simulink model "RO_Plantsimscape"  (R2020a)
settings: Solver=VariableStepAuto  StartTime=0.0  StopTime=100  RelTol=1e-3
libraries: sh_lib x108, fl_lib x76, nesl_utility x73, simulink x13
(part 4 of 4)

== system RO_Plantsimscape/PSOC8 ==
  E : Inport
  Hydraulic Flow Rate Sensor : fl_lib/Hydraulic/Hydraulic Sensors/Hydraulic Flow Rate Sensor
  PS-Simulink Converter2 : nesl_utility/PS-Simulink Converter  PhysicalDomain=network_engine_domain  SubClassName=ps_output  LeftPortType=input  RightPortType=output  PseudoPeriodic=off  Frequencies=[]  Unit=1  AffineConversion=off
  Pipe P : sh_lib/Low-Pressure Blocks/Resistive Pipe LP  cs_type=1  d_in=112.1660 mm  area=1e-04 m^2  D_h=0.0112 m  s_factor=64  length=8.1 m  length_ad=1 m  roughness=0.005 mm  Re_lam=2e+03  Re_turb=4e+03  elevation_A=45 m  elevation_B=45 m  g=9.80665 m/s^2  pressure_drop_specify=off  pressure_drop_priority=None  pressure_drop=0 Pa  pressure_drop_nominal_specify=off  pressure_drop_nominal_unit=Pa  pressure_drop_nominal_value=1  flow_rate_specify=off  flow_rate_priority=None  flow_rate=0 m^3/s  flow_rate_nominal_specify=off  flow_rate_nominal_unit=m^3/s  flow_rate_nominal_value=1
      settings: SourceProductBaseCode=SH  InternalSimscapePortConfiguration="{\"Bottom\":[],\"Left\":[{\"id\":\"A\",\"label\":\"A\",\"type\":\"foundation.hydraulic.hydraulic\"}],\"Right\":[{\"id\":\"B\",\"label\":\"B\",\"type\":\"foundation.hydraulic.hydraulic\"}],\"Top\":[]}"
  "Pneumatic Pump, Drive and Amplifier" : TransferFcn  Denominator=[0.1 1]
  Poppet Valve : sh_lib/Valves/Flow Control Valves/Poppet Valve  d_stem=0.01 m  cone_angle=120 deg  x_0=0 m  C_d=0.65  A_leak=1e-12 m^2  lam_spec=1  B_lam=0.999  Re_cr=10
      settings: SourceProductBaseCode=SH  InternalSimscapePortConfiguration="{\"Bottom\":[],\"Left\":[{\"id\":\"S\",\"label\":\"S\",\"type\":\"input\"},{\"id\":\"A\",\"label\":\"A\",\"type\":\"foundation.hydraulic.hydraulic\"}],\"Right\":[{\"id\":\"B\",\"label\":\"B\",\"type\":\"foundation.hydraulic.hydraulic\"}],\"Top\":[]}"
  Saturation : Saturate  UpperLimit=100  LowerLimit=0
  Scope : Scope
  Scope1 : Scope
  Simulink-PS Converter1 : nesl_utility/Simulink-PS Converter  PhysicalDomain=network_engine_domain  SubClassName=ps_input  LeftPortType=input  RightPortType=output  PseudoPeriodic=off  Frequencies=[]  NoiseDistribution=none  NoiseParameters=[]  Unit=1  AffineConversion=on  FilteringAndDerivatives=zero  SimscapeFilterOrder=1  InputFilterTimeConstant=.001  UdotUserProvided=0
  Valve Stiction : TransportDelay  DelayTime=0.5
  Out : PMIOPort  Side=Right
  In : PMIOPort  Port=2  Side=Left
  wires:
  E/1 -> "Pneumatic Pump, Drive and Amplifier"/1
  "Pneumatic Pump, Drive and Amplifier"/1 -> Valve Stiction/1
  PS-Simulink Converter2/1 -> Scope1/1
  Valve Stiction/1 -> Saturation/1
  Saturation/1 -> Scope/1, Simulink-PS Converter1/1
  connections:
  Simulink-PS Converter1/RConn1 -- Poppet Valve/LConn1
  In/RConn1 -- Poppet Valve/LConn2
  Hydraulic Flow Rate Sensor/RConn2 -- Out/RConn1
  Hydraulic Flow Rate Sensor/RConn1 -- PS-Simulink Converter2/LConn1
  Poppet Valve/RConn1 -- Pipe P/LConn1
  Hydraulic Flow Rate Sensor/LConn1 -- Pipe P/RConn1

== system RO_Plantsimscape/PSOC9 ==
  E : Inport
  Hydraulic Flow Rate Sensor : fl_lib/Hydraulic/Hydraulic Sensors/Hydraulic Flow Rate Sensor
  PS-Simulink Converter2 : nesl_utility/PS-Simulink Converter  PhysicalDomain=network_engine_domain  SubClassName=ps_output  LeftPortType=input  RightPortType=output  PseudoPeriodic=off  Frequencies=[]  Unit=1  AffineConversion=off
  Pipe P : sh_lib/Low-Pressure Blocks/Resistive Pipe LP  cs_type=1  d_in=112.1660 mm  area=1e-04 m^2  D_h=0.0112 m  s_factor=64  length=8.1 m  length_ad=1 m  roughness=0.005 mm  Re_lam=2e+03  Re_turb=4e+03  elevation_A=45 m  elevation_B=45 m  g=9.80665 m/s^2  pressure_drop_specify=off  pressure_drop_priority=None  pressure_drop=0 Pa  pressure_drop_nominal_specify=off  pressure_drop_nominal_unit=Pa  pressure_drop_nominal_value=1  flow_rate_specify=off  flow_rate_priority=None  flow_rate=0 m^3/s  flow_rate_nominal_specify=off  flow_rate_nominal_unit=m^3/s  flow_rate_nominal_value=1
      settings: SourceProductBaseCode=SH  InternalSimscapePortConfiguration="{\"Bottom\":[],\"Left\":[{\"id\":\"A\",\"label\":\"A\",\"type\":\"foundation.hydraulic.hydraulic\"}],\"Right\":[{\"id\":\"B\",\"label\":\"B\",\"type\":\"foundation.hydraulic.hydraulic\"}],\"Top\":[]}"
  "Pneumatic Pump, Drive and Amplifier" : TransferFcn  Denominator=[0.1 1]
  Poppet Valve : sh_lib/Valves/Flow Control Valves/Poppet Valve  d_stem=0.01 m  cone_angle=120 deg  x_0=0 m  C_d=0.65  A_leak=1e-12 m^2  lam_spec=1  B_lam=0.999  Re_cr=10
      settings: SourceProductBaseCode=SH  InternalSimscapePortConfiguration="{\"Bottom\":[],\"Left\":[{\"id\":\"S\",\"label\":\"S\",\"type\":\"input\"},{\"id\":\"A\",\"label\":\"A\",\"type\":\"foundation.hydraulic.hydraulic\"}],\"Right\":[{\"id\":\"B\",\"label\":\"B\",\"type\":\"foundation.hydraulic.hydraulic\"}],\"Top\":[]}"
  Saturation : Saturate  UpperLimit=100  LowerLimit=0
  Scope : Scope
  Scope1 : Scope
  Simulink-PS Converter1 : nesl_utility/Simulink-PS Converter  PhysicalDomain=network_engine_domain  SubClassName=ps_input  LeftPortType=input  RightPortType=output  PseudoPeriodic=off  Frequencies=[]  NoiseDistribution=none  NoiseParameters=[]  Unit=1  AffineConversion=on  FilteringAndDerivatives=zero  SimscapeFilterOrder=1  InputFilterTimeConstant=.001  UdotUserProvided=0
  Valve Stiction : TransportDelay  DelayTime=0.5
  Out : PMIOPort  Side=Right
  In : PMIOPort  Port=2  Side=Left
  wires:
  E/1 -> "Pneumatic Pump, Drive and Amplifier"/1
  "Pneumatic Pump, Drive and Amplifier"/1 -> Valve Stiction/1
  PS-Simulink Converter2/1 -> Scope1/1
  Valve Stiction/1 -> Saturation/1
  Saturation/1 -> Scope/1, Simulink-PS Converter1/1
  connections:
  Simulink-PS Converter1/RConn1 -- Poppet Valve/LConn1
  In/RConn1 -- Poppet Valve/LConn2
  Hydraulic Flow Rate Sensor/RConn2 -- Out/RConn1
  Hydraulic Flow Rate Sensor/RConn1 -- PS-Simulink Converter2/LConn1
  Poppet Valve/RConn1 -- Pipe P/LConn1
  Hydraulic Flow Rate Sensor/LConn1 -- Pipe P/RConn1

== system RO_Plantsimscape/Rain ==
  Centrifugal Pump : Subsystem
      mask Display: image('$imagefile'); % Use "Edit Image" on toolstrip to change.
  Constant4 : Constant  Value=3000
  Poppet Valve : sh_lib/Valves/Flow Control Valves/Poppet Valve  d_stem=1 m  cone_angle=120 deg  x_0=0 m  C_d=1  A_leak=1e-12 m^2  lam_spec=2  B_lam=0.999  Re_cr=2300
      settings: SourceProductBaseCode=SH  InternalSimscapePortConfiguration="{\"Bottom\":[],\"Left\":[{\"id\":\"S\",\"label\":\"S\",\"type\":\"input\"},{\"id\":\"A\",\"label\":\"A\",\"type\":\"foundation.hydraulic.hydraulic\"}],\"Right\":[{\"id\":\"B\",\"label\":\"B\",\"type\":\"foundation.hydraulic.hydraulic\"}],\"Top\":[]}"
  Rain : sh_lib/Low-Pressure Blocks/Constant Head Tank  press=1 Pa  fluid_level=10000 m  pipe_diam=0.02 m  loss_coeff=1.2  g=9.80665 m/s^2  volume_specify=on  volume_priority=High  volume=1000 m^3  volume_nominal_specify=off  volume_nominal_unit=m^3  volume_nominal_value=1
      settings: SourceProductBaseCode=SH  InternalSimscapePortConfiguration="{\"Bottom\":[],\"Left\":[],\"Right\":[{\"id\":\"V\",\"label\":\"V\",\"type\":\"output\"},{\"id\":\"T\",\"label\":\"T\",\"type\":\"foundation.hydraulic.hydraulic\"}],\"Top\":[]}"
  Simulink-PS Converter1 : nesl_utility/Simulink-PS Converter  PhysicalDomain=network_engine_domain  SubClassName=ps_input  LeftPortType=input  RightPortType=output  PseudoPeriodic=off  Frequencies=[]  NoiseDistribution=none  NoiseParameters=[]  Unit=1  AffineConversion=on  FilteringAndDerivatives=zero  SimscapeFilterOrder=1  InputFilterTimeConstant=.001  UdotUserProvided=0
  Sine Wave : Sin  Amplitude=10  Frequency=0.5  SampleTime=0
  Rain_ : PMIOPort  Side=Right
  wires:
  Sine Wave/1 -> Simulink-PS Converter1/1
  Constant4/1 -> Centrifugal Pump/1(f)
  connections:
  Poppet Valve/LConn1 -- Simulink-PS Converter1/RConn1
  Rain_/RConn1 -- Poppet Valve/RConn1
  Centrifugal Pump/LConn1 -- Rain/RConn2
  Centrifugal Pump/RConn1 -- Poppet Valve/LConn2

== system RO_Plantsimscape/Centrifugal Pump1/induction machine ==
  note: Voltage/Hz control
  note: TODO: Set the number of poles,
      | the induction machine's time constant and
      | the maximum rotor speed in rad/s
  f : Inport
  Induction Machine : TransferFcn  Denominator=[1 1]
  Induction speed : MATLAB Function  TreatAsAtomicUnit=on
  max/min speeds : Saturate  UpperLimit=100  LowerLimit=0
  w : Outport
  wires:
  f/1 -> Induction speed/1(f)
  Induction speed/1(w) -> Induction Machine/1
  max/min speeds/1 -> w/1
  Induction Machine/1 -> max/min speeds/1

== system RO_Plantsimscape/Centrifugal Pump2/induction machine ==
  note: Voltage/Hz control
  note: TODO: Set the number of poles,
      | the induction machine's time constant and
      | the maximum rotor speed in rad/s
  f : Inport
  Induction Machine : TransferFcn  Denominator=[1 1]
  Induction speed : MATLAB Function  TreatAsAtomicUnit=on
  max/min speeds : Saturate  UpperLimit=10000  LowerLimit=0
  w : Outport
  wires:
  f/1 -> Induction speed/1(f)
  Induction speed/1(w) -> Induction Machine/1
  max/min speeds/1 -> w/1
  Induction Machine/1 -> max/min speeds/1

== system RO_Plantsimscape/Centrifugal Pump3/induction machine ==
  note: Voltage/Hz control
  note: TODO: Set the number of poles,
      | the induction machine's time constant and
      | the maximum rotor speed in rad/s
  f : Inport
  Induction Machine : TransferFcn  Denominator=[1 1]
  Induction speed : MATLAB Function  TreatAsAtomicUnit=on
  max/min speeds : Saturate  UpperLimit=10000  LowerLimit=0
  w : Outport
  wires:
  f/1 -> Induction speed/1(f)
  Induction speed/1(w) -> Induction Machine/1
  max/min speeds/1 -> w/1
  Induction Machine/1 -> max/min speeds/1

== system RO_Plantsimscape/Centrifugal Pump4/induction machine ==
  note: Voltage/Hz control
  note: TODO: Set the number of poles,
      | the induction machine's time constant and
      | the maximum rotor speed in rad/s
  f : Inport
  Induction Machine : TransferFcn  Denominator=[1 1]
  Induction speed : MATLAB Function  TreatAsAtomicUnit=on
  max/min speeds : Saturate  UpperLimit=10000  LowerLimit=0
  w : Outport
  wires:
  f/1 -> Induction speed/1(f)
  Induction speed/1(w) -> Induction Machine/1
  max/min speeds/1 -> w/1
  Induction Machine/1 -> max/min speeds/1

== system RO_Plantsimscape/Centrifugal Pump5/induction machine ==
  note: Voltage/Hz control
  note: TODO: Set the number of poles,
      | the induction machine's time constant and
      | the maximum rotor speed in rad/s
  f : Inport
  Induction Machine : TransferFcn  Denominator=[1 1]
  Induction speed : MATLAB Function  TreatAsAtomicUnit=on
  max/min speeds : Saturate  UpperLimit=100  LowerLimit=0
  w : Outport
  wires:
  f/1 -> Induction speed/1(f)
  Induction speed/1(w) -> Induction Machine/1
  max/min speeds/1 -> w/1
  Induction Machine/1 -> max/min speeds/1

== system RO_Plantsimscape/Centrifugal Pump6/induction machine ==
  note: Voltage/Hz control
  note: TODO: Set the number of poles,
      | the induction machine's time constant and
      | the maximum rotor speed in rad/s
  f : Inport
  Induction Machine : TransferFcn  Denominator=[1 1]
  Induction speed : MATLAB Function  TreatAsAtomicUnit=on
  max/min speeds : Saturate  UpperLimit=100  LowerLimit=0
  w : Outport
  wires:
  f/1 -> Induction speed/1(f)
  Induction speed/1(w) -> Induction Machine/1
  max/min speeds/1 -> w/1
  Induction Machine/1 -> max/min speeds/1

== system RO_Plantsimscape/Centrifugal Pump7/induction machine ==
  note: Voltage/Hz control
  note: TODO: Set the number of poles,
      | the induction machine's time constant and
      | the maximum rotor speed in rad/s
  f : Inport
  Induction Machine : TransferFcn  Denominator=[1 1]
  Induction speed : MATLAB Function  TreatAsAtomicUnit=on
  max/min speeds : Saturate  UpperLimit=10000  LowerLimit=0
  w : Outport
  wires:
  f/1 -> Induction speed/1(f)
  Induction speed/1(w) -> Induction Machine/1
  max/min speeds/1 -> w/1
  Induction Machine/1 -> max/min speeds/1

== system RO_Plantsimscape/Centrifugal Pump8/induction machine ==
  note: Voltage/Hz control
  note: TODO: Set the number of poles,
      | the induction machine's time constant and
      | the maximum rotor speed in rad/s
  f : Inport
  Induction Machine : TransferFcn  Denominator=[1 1]
  Induction speed : MATLAB Function  TreatAsAtomicUnit=on
  max/min speeds : Saturate  UpperLimit=10000  LowerLimit=0
  w : Outport
  wires:
  f/1 -> Induction speed/1(f)
  Induction speed/1(w) -> Induction Machine/1
  max/min speeds/1 -> w/1
  Induction Machine/1 -> max/min speeds/1

== system RO_Plantsimscape/FRO1/Centrifugal Pump3 ==
  f : Inport
  Drive and Amplifier Dynamics : TransferFcn  Denominator=[0.1 1]
  Hydraulic Flow Rate Sensor : fl_lib/Hydraulic/Hydraulic Sensors/Hydraulic Flow Rate Sensor
  MRRef Pump 1 : fl_lib/Mechanical/Rotational Elements/Mechanical Rotational Reference
  PS-Simulink Converter2 : nesl_utility/PS-Simulink Converter  PhysicalDomain=network_engine_domain  SubClassName=ps_output  LeftPortType=input  RightPortType=output  PseudoPeriodic=off  Frequencies=[]  Unit=1  AffineConversion=off
  Pipe P : sh_lib/Low-Pressure Blocks/Resistive Pipe LP  cs_type=1  d_in=112.1660 mm  area=1e-04 m^2  D_h=0.0112 m  s_factor=64  length=8.1 m  length_ad=1 m  roughness=0.005 mm  Re_lam=2e+03  Re_turb=4e+03  elevation_A=45 m  elevation_B=45 m  g=9.80665 m/s^2  pressure_drop_specify=off  pressure_drop_priority=None  pressure_drop=0 Pa  pressure_drop_nominal_specify=off  pressure_drop_nominal_unit=Pa  pressure_drop_nominal_value=1  flow_rate_specify=off  flow_rate_priority=None  flow_rate=0 m^3/s  flow_rate_nominal_specify=off  flow_rate_nominal_unit=m^3/s  flow_rate_nominal_value=1
      settings: SourceProductBaseCode=SH  InternalSimscapePortConfiguration="{\"Bottom\":[],\"Left\":[{\"id\":\"A\",\"label\":\"A\",\"type\":\"foundation.hydraulic.hydraulic\"}],\"Right\":[{\"id\":\"B\",\"label\":\"B\",\"type\":\"foundation.hydraulic.hydraulic\"}],\"Top\":[]}"
  Pump 1 : sh_lib/Pumps and Motors/Centrifugal Pump  mdl_type=2  c_1=326.8 Pa/(kg/m^3)  c_2=3.104e+04 Pa*s/kg  c_3=1.097e+07 Pa*s^2/(kg*m^3)  c_4=2.136e+05 Pa*s^2/(kg*m^3)  c_f=0.8  design_del=130 lpm  ref_velocity=1.77e+03 rpm  ref_density=1000 kg/m^3  leak_resistance=1e+8 Pa/(m^3/s)  T_const=0.1 N*m  trq_press_coeff=1e-6 N*m/Pa  pump_del_1D="[0    0.0032    0.0063    0.0095    0.0126    0.0158] m^3/s"  press_diff_1D="[4.4851    4.3655    4.1413    3.7376    2.9901    1.7940] bar"  pump_del_power_1D="[0    0.0032    0.0063    0.0095    0.0126    0.0158] m^3/s"  power_1D="[0\t2116.60000000000\t3727.20000000000\t4734.30000000000\t5232.70000000000\t4360.90000000000] W"  pump_vel_2D="[  3.2e+03 3.3e+03 3.4e+03 3.5e+03 ] rpm"  pump_del_2D="[  0 50 100 150 200 250 300 350 ] lpm"  press_diff_2D="[  8.3 8.8 9.3 9.9 ; 7.8 8.3 8.8 9.4 ; 7.2 7.6 8.2 8.7 ; 6.5 7 7.5 8 ; 5.6 6.1 6.6 7.1 ; 4.7 5.2 5.7 6.2 ; 3.4 4 4.4 4.9 ; 2.3 2.7 3.4 3.6 ; ] bar"  pump_del_power_2D="[  0 50 100 150 200 250 300 350 ] lpm"  power_2D="[  1.223e+03 1.341e+03 1.467e+03 1.6e+03 ; 1.414e+03 1.551e+03 1.696e+03 1.85e+03 ; 1.636e+03 1.794e+03 1.962e+03 2.14e+03 ; 1.941e+03 2.129e+03 2.326e+03 2.54e+03 ; 2.224e+03 2.439e+03 2.66e+03 2.91e+03 ; 2.453e+03 2.691e+03 2.947e+03 3.21e+03 ; 2.757e+03 3.024e+03 3.307e+03 3.608e+03 ; 2.945e+03 3.23e+03 3.533e+03 3.854e+03 ; ] W"  omega_threshold=1e-9 rad/s  interp_method=2  extrap_method=1
      settings: SourceProductBaseCode=SH  InternalSimscapePortConfiguration="{\"Bottom\":[],\"Left\":[{\"id\":\"S\",\"label\":\"S\",\"type\":\"foundation.mechanical.rotational.rotational\"}],\"Right\":[{\"id\":\"P\",\"label\":\"P\",\"type\":\"foundation.hydraulic.hydraulic\"},{\"id\":\"T\",\"label\":\"T\",\"type\":\"foundation.hydraulic.hydraulic\"}],\"Top\":[]}"
  Scope : Scope
  Simulink-PS Converter1 : nesl_utility/Simulink-PS Converter  PhysicalDomain=network_engine_domain  SubClassName=ps_input  LeftPortType=input  RightPortType=output  PseudoPeriodic=off  Frequencies=[]  NoiseDistribution=none  NoiseParameters=[]  Unit=rpm  AffineConversion=off  FilteringAndDerivatives=zero  SimscapeFilterOrder=1  InputFilterTimeConstant=.001  UdotUserProvided=0
  Velocity Source Pump 1 : fl_lib/Mechanical/Mechanical Sources/Ideal Angular Velocity Source
  induction machine : Subsystem
  inletT : PMIOPort  Side=Left
  outletT : PMIOPort  Port=2  Side=Right
  wires:
  f/1 -> Drive and Amplifier Dynamics/1
  induction machine/1(w) -> Simulink-PS Converter1/1
  Drive and Amplifier Dynamics/1 -> induction machine/1(f)
  PS-Simulink Converter2/1 -> Scope/1
  connections:
  Velocity Source Pump 1/LConn1 -- Pump 1/LConn1
  MRRef Pump 1/LConn1 -- Velocity Source Pump 1/RConn2
  inletT/RConn1 -- Pump 1/RConn2
  Pipe P/LConn1 -- Pump 1/RConn1
  Simulink-PS Converter1/RConn1 -- Velocity Source Pump 1/RConn1
  Pipe P/RConn1 -- Hydraulic Flow Rate Sensor/LConn1
  Hydraulic Flow Rate Sensor/RConn2 -- outletT/RConn1
  PS-Simulink Converter2/LConn1 -- Hydraulic Flow Rate Sensor/RConn1

== system RO_Plantsimscape/FRO3/Centrifugal Pump3 ==
  f : Inport
  Drive and Amplifier Dynamics : TransferFcn  Denominator=[0.1 1]
  Hydraulic Flow Rate Sensor : fl_lib/Hydraulic/Hydraulic Sensors/Hydraulic Flow Rate Sensor
  MRRef Pump 1 : fl_lib/Mechanical/Rotational Elements/Mechanical Rotational Reference
  PS-Simulink Converter2 : nesl_utility/PS-Simulink Converter  PhysicalDomain=network_engine_domain  SubClassName=ps_output  LeftPortType=input  RightPortType=output  PseudoPeriodic=off  Frequencies=[]  Unit=1  AffineConversion=off
  Pipe P : sh_lib/Low-Pressure Blocks/Resistive Pipe LP  cs_type=1  d_in=112.1660 mm  area=1e-04 m^2  D_h=0.0112 m  s_factor=64  length=8.1 m  length_ad=1 m  roughness=0.005 mm  Re_lam=2e+03  Re_turb=4e+03  elevation_A=45 m  elevation_B=45 m  g=9.80665 m/s^2  pressure_drop_specify=off  pressure_drop_priority=None  pressure_drop=0 Pa  pressure_drop_nominal_specify=off  pressure_drop_nominal_unit=Pa  pressure_drop_nominal_value=1  flow_rate_specify=off  flow_rate_priority=None  flow_rate=0 m^3/s  flow_rate_nominal_specify=off  flow_rate_nominal_unit=m^3/s  flow_rate_nominal_value=1
      settings: SourceProductBaseCode=SH  InternalSimscapePortConfiguration="{\"Bottom\":[],\"Left\":[{\"id\":\"A\",\"label\":\"A\",\"type\":\"foundation.hydraulic.hydraulic\"}],\"Right\":[{\"id\":\"B\",\"label\":\"B\",\"type\":\"foundation.hydraulic.hydraulic\"}],\"Top\":[]}"
  Pump 1 : sh_lib/Pumps and Motors/Centrifugal Pump  mdl_type=2  c_1=326.8 Pa/(kg/m^3)  c_2=3.104e+04 Pa*s/kg  c_3=1.097e+07 Pa*s^2/(kg*m^3)  c_4=2.136e+05 Pa*s^2/(kg*m^3)  c_f=0.8  design_del=130 lpm  ref_velocity=1.77e+03 rpm  ref_density=1000 kg/m^3  leak_resistance=1e+8 Pa/(m^3/s)  T_const=0.1 N*m  trq_press_coeff=1e-6 N*m/Pa  pump_del_1D="[0    0.0032    0.0063    0.0095    0.0126    0.0158] m^3/s"  press_diff_1D="[4.4851    4.3655    4.1413    3.7376    2.9901    1.7940] bar"  pump_del_power_1D="[0    0.0032    0.0063    0.0095    0.0126    0.0158] m^3/s"  power_1D="[0\t2116.60000000000\t3727.20000000000\t4734.30000000000\t5232.70000000000\t4360.90000000000] W"  pump_vel_2D="[  3.2e+03 3.3e+03 3.4e+03 3.5e+03 ] rpm"  pump_del_2D="[  0 50 100 150 200 250 300 350 ] lpm"  press_diff_2D="[  8.3 8.8 9.3 9.9 ; 7.8 8.3 8.8 9.4 ; 7.2 7.6 8.2 8.7 ; 6.5 7 7.5 8 ; 5.6 6.1 6.6 7.1 ; 4.7 5.2 5.7 6.2 ; 3.4 4 4.4 4.9 ; 2.3 2.7 3.4 3.6 ; ] bar"  pump_del_power_2D="[  0 50 100 150 200 250 300 350 ] lpm"  power_2D="[  1.223e+03 1.341e+03 1.467e+03 1.6e+03 ; 1.414e+03 1.551e+03 1.696e+03 1.85e+03 ; 1.636e+03 1.794e+03 1.962e+03 2.14e+03 ; 1.941e+03 2.129e+03 2.326e+03 2.54e+03 ; 2.224e+03 2.439e+03 2.66e+03 2.91e+03 ; 2.453e+03 2.691e+03 2.947e+03 3.21e+03 ; 2.757e+03 3.024e+03 3.307e+03 3.608e+03 ; 2.945e+03 3.23e+03 3.533e+03 3.854e+03 ; ] W"  omega_threshold=1e-9 rad/s  interp_method=2  extrap_method=1
      settings: SourceProductBaseCode=SH  InternalSimscapePortConfiguration="{\"Bottom\":[],\"Left\":[{\"id\":\"S\",\"label\":\"S\",\"type\":\"foundation.mechanical.rotational.rotational\"}],\"Right\":[{\"id\":\"P\",\"label\":\"P\",\"type\":\"foundation.hydraulic.hydraulic\"},{\"id\":\"T\",\"label\":\"T\",\"type\":\"foundation.hydraulic.hydraulic\"}],\"Top\":[]}"
  Scope : Scope
  Simulink-PS Converter1 : nesl_utility/Simulink-PS Converter  PhysicalDomain=network_engine_domain  SubClassName=ps_input  LeftPortType=input  RightPortType=output  PseudoPeriodic=off  Frequencies=[]  NoiseDistribution=none  NoiseParameters=[]  Unit=rpm  AffineConversion=off  FilteringAndDerivatives=zero  SimscapeFilterOrder=1  InputFilterTimeConstant=.001  UdotUserProvided=0
  Velocity Source Pump 1 : fl_lib/Mechanical/Mechanical Sources/Ideal Angular Velocity Source
  induction machine : Subsystem
  inletT : PMIOPort  Side=Left
  outletT : PMIOPort  Port=2  Side=Right
  wires:
  f/1 -> Drive and Amplifier Dynamics/1
  induction machine/1(w) -> Simulink-PS Converter1/1
  Drive and Amplifier Dynamics/1 -> induction machine/1(f)
  PS-Simulink Converter2/1 -> Scope/1
  connections:
  Velocity Source Pump 1/LConn1 -- Pump 1/LConn1
  MRRef Pump 1/LConn1 -- Velocity Source Pump 1/RConn2
  inletT/RConn1 -- Pump 1/RConn2
  Pipe P/LConn1 -- Pump 1/RConn1
  Simulink-PS Converter1/RConn1 -- Velocity Source Pump 1/RConn1
  Pipe P/RConn1 -- Hydraulic Flow Rate Sensor/LConn1
  Hydraulic Flow Rate Sensor/RConn2 -- outletT/RConn1
  PS-Simulink Converter2/LConn1 -- Hydraulic Flow Rate Sensor/RConn1

== system RO_Plantsimscape/Rain/Centrifugal Pump ==
  f : Inport
  Drive and Amplifier Dynamics : TransferFcn  Denominator=[0.1 1]
  Hydraulic Flow Rate Sensor : fl_lib/Hydraulic/Hydraulic Sensors/Hydraulic Flow Rate Sensor
  MRRef Pump 1 : fl_lib/Mechanical/Rotational Elements/Mechanical Rotational Reference
  PS-Simulink Converter2 : nesl_utility/PS-Simulink Converter  PhysicalDomain=network_engine_domain  SubClassName=ps_output  LeftPortType=input  RightPortType=output  PseudoPeriodic=off  Frequencies=[]  Unit=1  AffineConversion=off
  Pump 1 : sh_lib/Pumps and Motors/Centrifugal Pump  mdl_type=1  c_1=500 Pa/(kg/m^3)  c_2=3.104e+04 Pa*s/kg  c_3=1.097e+07 Pa*s^2/(kg*m^3)  c_4=2.136e+05 Pa*s^2/(kg*m^3)  c_f=0.8  design_del=1000 lpm  ref_velocity=2000 rpm  ref_density=1000 kg/m^3  leak_resistance=1e+8 Pa/(m^3/s)  T_const=0.1 N*m  trq_press_coeff=1e-6 N*m/Pa  pump_del_1D="[0    0.0032    0.0063    0.0095    0.0126    0.0158] m^3/s"  press_diff_1D="[4.4851    4.3655    4.1413    3.7376    2.9901    1.7940] bar"  pump_del_power_1D="[0    0.0032    0.0063    0.0095    0.0126    0.0158] m^3/s"  power_1D="[0\t2116.60000000000\t3727.20000000000\t4734.30000000000\t5232.70000000000\t4360.90000000000] W"  pump_vel_2D="[  3.2e+03 3.3e+03 3.4e+03 3.5e+03 ] rpm"  pump_del_2D="[  0 50 100 150 200 250 300 350 ] lpm"  press_diff_2D="[  8.3 8.8 9.3 9.9 ; 7.8 8.3 8.8 9.4 ; 7.2 7.6 8.2 8.7 ; 6.5 7 7.5 8 ; 5.6 6.1 6.6 7.1 ; 4.7 5.2 5.7 6.2 ; 3.4 4 4.4 4.9 ; 2.3 2.7 3.4 3.6 ; ] bar"  pump_del_power_2D="[  0 50 100 150 200 250 300 350 ] lpm"  power_2D="[  1.223e+03 1.341e+03 1.467e+03 1.6e+03 ; 1.414e+03 1.551e+03 1.696e+03 1.85e+03 ; 1.636e+03 1.794e+03 1.962e+03 2.14e+03 ; 1.941e+03 2.129e+03 2.326e+03 2.54e+03 ; 2.224e+03 2.439e+03 2.66e+03 2.91e+03 ; 2.453e+03 2.691e+03 2.947e+03 3.21e+03 ; 2.757e+03 3.024e+03 3.307e+03 3.608e+03 ; 2.945e+03 3.23e+03 3.533e+03 3.854e+03 ; ] W"  omega_threshold=1e-9 rad/s  interp_method=2  extrap_method=1
      settings: SourceProductBaseCode=SH  InternalSimscapePortConfiguration="{\"Bottom\":[],\"Left\":[{\"id\":\"S\",\"label\":\"S\",\"type\":\"foundation.mechanical.rotational.rotational\"}],\"Right\":[{\"id\":\"P\",\"label\":\"P\",\"type\":\"foundation.hydraulic.hydraulic\"},{\"id\":\"T\",\"label\":\"T\",\"type\":\"foundation.hydraulic.hydraulic\"}],\"Top\":[]}"
  Scope : Scope
  Simulink-PS Converter1 : nesl_utility/Simulink-PS Converter  PhysicalDomain=network_engine_domain  SubClassName=ps_input  LeftPortType=input  RightPortType=output  PseudoPeriodic=off  Frequencies=[]  NoiseDistribution=none  NoiseParameters=[]  Unit=rpm  AffineConversion=off  FilteringAndDerivatives=zero  SimscapeFilterOrder=1  InputFilterTimeConstant=.001  UdotUserProvided=0
  Velocity Source Pump 1 : fl_lib/Mechanical/Mechanical Sources/Ideal Angular Velocity Source
  induction machine : Subsystem
  inletT : PMIOPort  Side=Left
  outletT : PMIOPort  Port=2  Side=Right
  wires:
  f/1 -> Drive and Amplifier Dynamics/1
  induction machine/1(w) -> Simulink-PS Converter1/1
  Drive and Amplifier Dynamics/1 -> induction machine/1(f)
  PS-Simulink Converter2/1 -> Scope/1
  connections:
  Velocity Source Pump 1/LConn1 -- Pump 1/LConn1
  MRRef Pump 1/LConn1 -- Velocity Source Pump 1/RConn2
  inletT/RConn1 -- Pump 1/RConn2
  Simulink-PS Converter1/RConn1 -- Velocity Source Pump 1/RConn1
  Pump 1/RConn1 -- Hydraulic Flow Rate Sensor/LConn1
  Hydraulic Flow Rate Sensor/RConn2 -- outletT/RConn1
  PS-Simulink Converter2/LConn1 -- Hydraulic Flow Rate Sensor/RConn1

== system RO_Plantsimscape/FRO1/Centrifugal Pump3/induction machine ==
  note: Voltage/Hz control
  note: TODO: Set the number of poles,
      | the induction machine's time constant and
      | the maximum rotor speed in rad/s
  f : Inport
  Induction Machine : TransferFcn  Denominator=[1 1]
  Induction speed : MATLAB Function  TreatAsAtomicUnit=on
  max/min speeds : Saturate  UpperLimit=100  LowerLimit=0
  w : Outport
  wires:
  f/1 -> Induction speed/1(f)
  Induction speed/1(w) -> Induction Machine/1
  max/min speeds/1 -> w/1
  Induction Machine/1 -> max/min speeds/1

== system RO_Plantsimscape/FRO3/Centrifugal Pump3/induction machine ==
  note: Voltage/Hz control
  note: TODO: Set the number of poles,
      | the induction machine's time constant and
      | the maximum rotor speed in rad/s
  f : Inport
  Induction Machine : TransferFcn  Denominator=[1 1]
  Induction speed : MATLAB Function  TreatAsAtomicUnit=on
  max/min speeds : Saturate  UpperLimit=100  LowerLimit=0
  w : Outport
  wires:
  f/1 -> Induction speed/1(f)
  Induction speed/1(w) -> Induction Machine/1
  max/min speeds/1 -> w/1
  Induction Machine/1 -> max/min speeds/1

== system RO_Plantsimscape/Rain/Centrifugal Pump/induction machine ==
  note: Voltage/Hz control
  note: TODO: Set the number of poles,
      | the induction machine's time constant and
      | the maximum rotor speed in rad/s
  f : Inport
  Induction Machine : TransferFcn  Denominator=[1 1]
  Induction speed : MATLAB Function  TreatAsAtomicUnit=on
  max/min speeds : Saturate  UpperLimit=10000  LowerLimit=0
  w : Outport
  wires:
  f/1 -> Induction speed/1(f)
  Induction speed/1(w) -> Induction Machine/1
  max/min speeds/1 -> w/1
  Induction Machine/1 -> max/min speeds/1

== matlab function RO_Plantsimscape/Rain/Centrifugal Pump/induction machine/Induction speed ==
  data: f input; w output
function w = fcn(f)
%w speed in rad/s
P=4; %number of poles of the induction machine
w=120*f/P; %speed in rpm
w=w*2*pi/60; %speed in rad/s

== matlab function RO_Plantsimscape/FRO1/Centrifugal Pump3/induction machine/Induction speed ==
  data: f input; w output
function w = fcn(f)
%w speed in rad/s
P=4; %number of poles of the induction machine
w=120*f/P; %speed in rpm
w=w*2*pi/60; %speed in rad/s

== matlab function RO_Plantsimscape/FRO3/Centrifugal Pump3/induction machine/Induction speed ==
  data: f input; w output
function w = fcn(f)
%w speed in rad/s
P=4; %number of poles of the induction machine
w=120*f/P; %speed in rpm
w=w*2*pi/60; %speed in rad/s

== matlab function RO_Plantsimscape/Centrifugal Pump2/induction machine/Induction speed ==
  data: f input; w output
function w = fcn(f)
%w speed in rad/s
P=4; %number of poles of the induction machine
w=120*f/P; %speed in rpm
w=w*2*pi/60; %speed in rad/s

== matlab function RO_Plantsimscape/Centrifugal Pump3/induction machine/Induction speed ==
  data: f input; w output
function w = fcn(f)
%w speed in rad/s
P=4; %number of poles of the induction machine
w=120*f/P; %speed in rpm
w=w*2*pi/60; %speed in rad/s

== matlab function RO_Plantsimscape/Centrifugal Pump4/induction machine/Induction speed ==
  data: f input; w output
function w = fcn(f)
%w speed in rad/s
P=4; %number of poles of the induction machine
w=120*f/P; %speed in rpm
w=w*2*pi/60; %speed in rad/s

== matlab function RO_Plantsimscape/Centrifugal Pump5/induction machine/Induction speed ==
  data: f input; w output
function w = fcn(f)
%w speed in rad/s
P=4; %number of poles of the induction machine
w=120*f/P; %speed in rpm
w=w*2*pi/60; %speed in rad/s

== matlab function RO_Plantsimscape/Centrifugal Pump6/induction machine/Induction speed ==
  data: f input; w output
function w = fcn(f)
%w speed in rad/s
P=4; %number of poles of the induction machine
w=120*f/P; %speed in rpm
w=w*2*pi/60; %speed in rad/s

== matlab function RO_Plantsimscape/Centrifugal Pump7/induction machine/Induction speed ==
  data: f input; w output
function w = fcn(f)
%w speed in rad/s
P=4; %number of poles of the induction machine
w=120*f/P; %speed in rpm
w=w*2*pi/60; %speed in rad/s

== matlab function RO_Plantsimscape/Centrifugal Pump8/induction machine/Induction speed ==
  data: f input; w output
function w = fcn(f)
%w speed in rad/s
P=4; %number of poles of the induction machine
w=120*f/P; %speed in rpm
w=w*2*pi/60; %speed in rad/s

== matlab function RO_Plantsimscape/Centrifugal Pump1/induction machine/Induction speed ==
  data: f input; w output
function w = fcn(f)
%w speed in rad/s
P=4; %number of poles of the induction machine
w=120*f/P; %speed in rpm
w=w*2*pi/60; %speed in rad/s
